simulink model "imukalmanfilter"  (R2023a)
settings: Solver=FixedStepAuto  StartTime=0.0  StopTime=inf  RelTol=1e-3
undefined symbols (not defined in the file or in its folder): DiscIntNeverNeededParam
libraries: matrix_library x3, arduinosensorlib x1
settings Model: ExtModeTrigDuration=2  Creator=82108  LastModifiedBy=admin
settings OptimizationCC: EnhancedBackFolding=on  PassReuseOutputArgsAs=Individual arguments  ZeroExternalMemoryAtStartup=off  ZeroInternalMemoryAtStartup=off  MaxStackSize=64  OptimizeBlockOrder=speed  DifferentSizesBufferReuse=on  OptimizationCustomize=off  EfficientTunableParamExpr=on
settings DebuggingCC: ParameterTunabilityLossMsg=error
settings HardwareCC: ProdBitPerInt=16  ProdBitPerPointer=16  ProdBitPerSizeT=16  ProdBitPerPtrDiffT=16  ProdLargestAtomicFloat=None  ProdWordSize=8  ProdHWDeviceType=Atmel->AVR
settings SFSimCC: MATLABDynamicMemAlloc=off
settings RTWCC: Description=Embedded Coder  SystemTargetFile=ert.tlc  HardwareBoard=Arduino Uno  TemplateMakefile=ert_default_tmf  Toolchain=Arduino AVR
settings CodeAppCC: ForceParamTrailComments=on  IgnoreCustomStorageClasses=off  OperatorAnnotations=on  SimulinkDataObjDesc=on  SFDataObjDesc=on  InsertBlockDesc=on
settings ERTTargetCC: SupportContinuousTime=on  SupportVariableSizeSignals=on  ExtModeTransport=3  ExtModeStaticAlloc=on  ExtModeAutomaticAllocSize=off  ExtModeStaticAllocSize=250  ExtModeMexFile=ext_xcp  ExtModeIntrfLevel=Level2 - Open

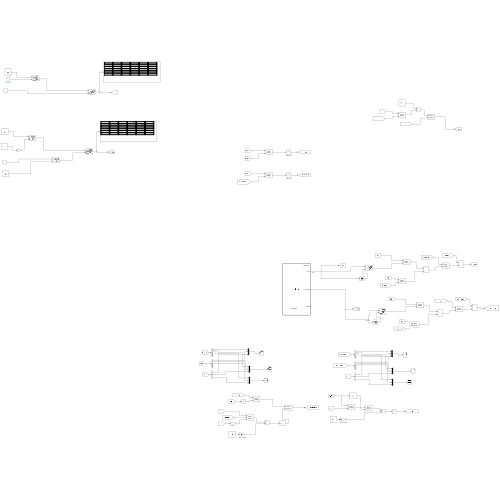
[thumbnail: Simulink's stored preview of the top-level diagram]
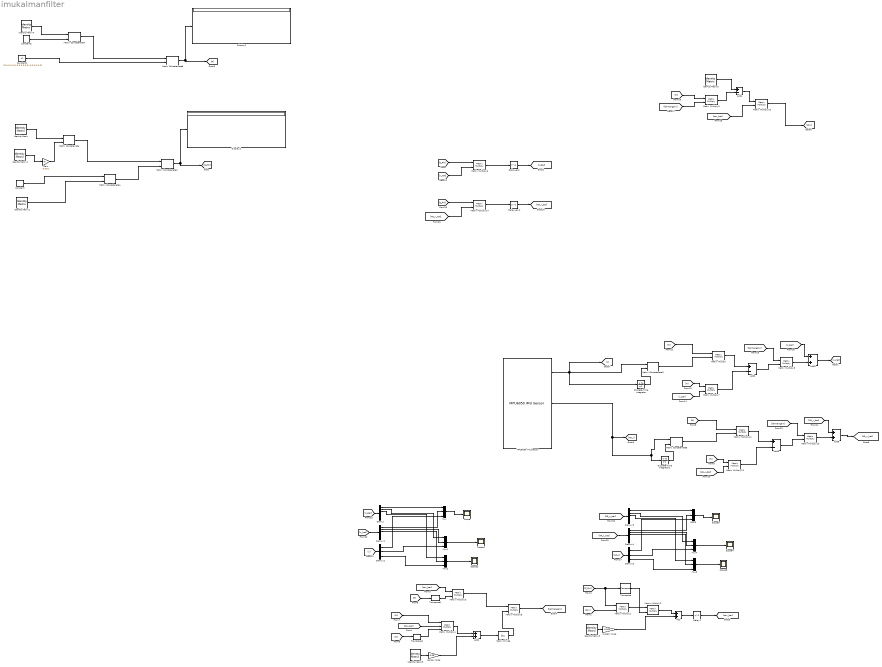
== system imukalmanfilter ==
  Add{,1,3,6} (4 alike) : Sum
  Add2 : Sum  Inputs=+-
  Add4 : Sum  Inputs=+-
  Add5 : Sum  Inputs=+-
  Constant : Constant  Value=[0 0 0; 0 0 0; 0 0 0]
  Constant1 : Constant  Value=[0 0 0 0 0 0; 0 0 0 0 0 0; 0 0 0 0 0 0]
  Constant2 : Constant  Value=[0 0 0; 0 0 0; 0 0 0]
  Delay1 : Delay  DelayLength=1
  Delay_acc : Delay  DelayLength=1  InitialCondition=[0; 0; 0; 0; 0;0]
  Delay_gyro : Delay  DelayLength=1
  Demux{,1,3..4} (4 alike) : Demux  Outputs=6
  Demux2 : Demux  Outputs=3
  Demux5 : Demux  Outputs=3
  Discrete-Time Integrator : DiscreteIntegrator  SampleTime=-1  ICPrevOutput=DiscIntNeverNeededParam  ICPrevScaledInput=DiscIntNeverNeededParam
  Discrete-Time Integrator1 : DiscreteIntegrator  SampleTime=-1  ICPrevOutput=DiscIntNeverNeededParam  ICPrevScaledInput=DiscIntNeverNeededParam
  Display1 : Display
  Display2 : Display
  Gain : Gain  Gain=-0.001
  IdentityMatrix{,1..2,4} (4 alike) : IdentityMatrix  OutputDimensions=3
  IdentityMatrix3 : IdentityMatrix  OutputDimensions=6
  IdentityMatrix5 : IdentityMatrix  OutputDimensions=6
  IdentityMatrix6 : IdentityMatrix  OutputDimensions=6
  MPU6050 IMU Sensor : arduinosensorlib/MPU6050 IMU Sensor  SlaveAddress=0x68  Accel=on  AngularRate=on  Temperature=off  Status=on  Timestamp=off  EulerAngles=off  Quat=off  AccelRange=2G  GyroRange=250 dps  DmpOdr=200 Hz  Dlpf=Accelerometer: 184Hz, Gyroscope: 188Hz  spf=1  SampleTime=0.001  QueueSizeFactor=1
  Matrix Concatenate : Concatenate  Mode=Multidimensional array  ConcatenateDimension=2
  Matrix Concatenate1 : Concatenate  Mode=Multidimensional array  ConcatenateDimension=2
  Matrix Concatenate{2..3,5..6} (4 alike) : Concatenate  Mode=Multidimensional array
  Matrix Concatenate4 : Concatenate  Mode=Multidimensional array  ConcatenateDimension=2
  Matrix Divide : Product  Inputs=/  Multiplication=Matrix(*)
  Matrix Multiply{,1..3,5..14} (14 alike) : Product  Multiplication=Matrix(*)
  Matrix Multiply4 : Product  Inputs=3  Multiplication=Matrix(*)
  Mux{,1..5} (6 alike) : Mux  Inputs=3
  Scope{,1..5} (6 alike) : Scope
  Transpose : matrix_library/Transpose
  Transpose1 : matrix_library/Transpose
  Transpose2 : matrix_library/Transpose
  sensor noise : Gain  Gain=0.08
  system noise : Gain  Gain=0.001
  wires:
  IdentityMatrix/1 -> Matrix Concatenate/1
  IdentityMatrix1/1 -> Gain/1
  Matrix Concatenate/1 -> Matrix Concatenate2/1
  Gain/1 -> Matrix Concatenate/2
  IdentityMatrix2/1 -> Matrix Concatenate1/2
  Constant/1 -> Matrix Concatenate1/1
  Matrix Concatenate1/1 -> Matrix Concatenate2/2
  Matrix Concatenate2/1 -> Display2/1, [C_Phi]
  [C_Phi] -> Matrix Multiply1/1, Transpose/1
  [cov] -> Matrix Multiply1/2
  Transpose/1 -> Matrix Multiply2/2
  Matrix Multiply1/1 -> Matrix Multiply2/1
  IdentityMatrix3/1 -> system noise/1
  Matrix Multiply2/1 -> Add/1
  Add/1 -> Delay1/1
  MPU6050 IMU Sensor/1 -> Matrix Concatenate3/1, Discrete-Time Integrator/1, [x]  "x_now"
  Discrete-Time Integrator/1 -> Matrix Concatenate3/2
  Matrix Concatenate3/1 -> Matrix Multiply/2
  Delay1/1 -> [cov_bar]
  Constant2/1 -> Matrix Concatenate4/2
  Matrix Concatenate4/1 -> Matrix Concatenate6/1
  Matrix Concatenate6/1 -> Display1/1, [H]
  IdentityMatrix4/1 -> Matrix Concatenate4/1
  Constant1/1 -> Matrix Concatenate6/2
  [H] -> Transpose1/1
  [cov_bar] -> Matrix Multiply3/1
  Transpose1/1 -> Matrix Multiply3/2
  [H] -> Transpose2/1
  [H] -> Matrix Multiply4/1
  [cov_bar] -> Matrix Multiply4/2
  Transpose2/1 -> Matrix Multiply4/3
  IdentityMatrix5/1 -> sensor noise/1
  Matrix Multiply4/1 -> Add1/1
  Add1/1 -> Matrix Divide/1
  Matrix Divide/1 -> Matrix Multiply5/2
  Matrix Multiply3/1 -> Matrix Multiply5/1
  Matrix Multiply5/1 -> [kalmangain]
  [H] -> Matrix Multiply/1
  Matrix Multiply6/1 -> Delay_acc/1
  Delay_acc/1 -> [x_bar]
  [C_Phi] -> Matrix Multiply6/1
  [x_hat] -> Matrix Multiply6/2
  Matrix Multiply/1 -> Add2/1
  [H] -> Matrix Multiply7/1
  [x_bar] -> Matrix Multiply7/2
  Matrix Multiply7/1 -> Add2/2
  [kalmangain] -> Matrix Multiply8/1
  Add2/1 -> Matrix Multiply8/2
  [x_bar] -> Add3/1
  Matrix Multiply8/1 -> Add3/2
  Add3/1 -> [x_hat]
  [H] -> Matrix Multiply9/1
  [kalmangain] -> Matrix Multiply9/2
  IdentityMatrix6/1 -> Add4/1
  Matrix Multiply9/1 -> Add4/2
  Add4/1 -> Matrix Multiply10/1
  [cov_bar] -> Matrix Multiply10/2
  Matrix Multiply10/1 -> [cov]
  Mux/1 -> Scope/1
  [x_bar] -> Demux/1
  [x_hat] -> Demux1/1
  [x] -> Demux2/1
  Mux1/1 -> Scope1/1
  Demux/1 -> Mux/1
  Demux1/1 -> Mux/2
  Demux2/1 -> Mux/3
  Demux/2 -> Mux1/1
  Demux1/2 -> Mux1/2
  Demux2/2 -> Mux1/3
  Demux/3 -> Mux2/1
  Demux1/3 -> Mux2/2
  Demux2/3 -> Mux2/3
  Mux2/1 -> Scope2/1
  Matrix Multiply11/1 -> Add5/1
  Add6/1 -> [AR_x_hat]
  [kalmangain] -> Matrix Multiply13/1
  Add5/1 -> Matrix Multiply13/2
  [H] -> Matrix Multiply12/1
  Matrix Multiply13/1 -> Add6/2
  Matrix Multiply12/1 -> Add5/2
  [AR_x_bar] -> Add6/1
  MPU6050 IMU Sensor/2 -> Matrix Concatenate5/1, Discrete-Time Integrator1/1, [AR_x]  "x_now_AR"
  [H] -> Matrix Multiply11/1
  [AR_x_bar] -> Matrix Multiply12/2
  Discrete-Time Integrator1/1 -> Matrix Concatenate5/2
  Matrix Concatenate5/1 -> Matrix Multiply11/2
  Delay_gyro/1 -> [AR_x_bar]
  Matrix Multiply14/1 -> Delay_gyro/1
  [AR_x_hat] -> Matrix Multiply14/2
  [C_Phi] -> Matrix Multiply14/1
  [AR_x_hat] -> Demux4/1
  Demux4/3 -> Mux5/2
  Mux5/1 -> Scope5/1
  Demux3/3 -> Mux5/1
  [AR_x_bar] -> Demux3/1
  Demux5/1 -> Mux3/3
  Demux3/2 -> Mux4/1
  [AR_x] -> Demux5/1
  Demux3/1 -> Mux3/1
  Demux4/1 -> Mux3/2
  Demux5/2 -> Mux4/3
  Demux4/2 -> Mux4/2
  Demux5/3 -> Mux5/3
  Mux4/1 -> Scope4/1
  Mux3/1 -> Scope3/1
  system noise/1 -> Add/2
  sensor noise/1 -> Add1/2
